simulink model "satellite"  (R2018b)
settings: Solver=VariableStepAuto  StartTime=0.0  StopTime=10.0  RelTol=1e-3
settings Model: Creator=carlos  LastModifiedBy=carlos

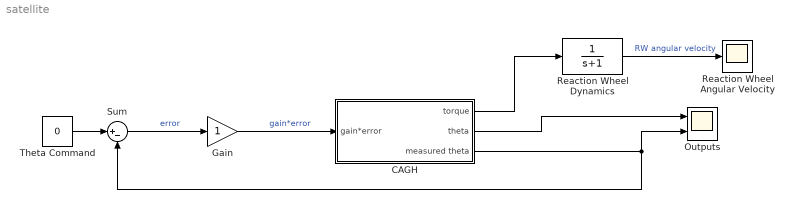
== system satellite ==
  CAGH : Subsystem
  Gain : Gain
  Outputs : Scope  NumInputPorts=2
  Reaction Wheel Angular Velocity : Scope
  Reaction Wheel Dynamics : TransferFcn  Denominator=[1 1]
  Sum : Sum  Inputs=|+-
  "Theta Command " : Constant  Value=0
  wires:
  "Theta Command "/1 -> Sum/1
  Sum/1 -> Gain/1  "error"
  Reaction Wheel Dynamics/1 -> Reaction Wheel Angular Velocity/1  "RW angular velocity"
  CAGH/3(measured theta) -> Outputs/2, Sum/2
  Gain/1 -> CAGH/1(gain*error)  "gain*error"
  CAGH/1(torque) -> Reaction Wheel Dynamics/1
  CAGH/2(theta) -> Outputs/1

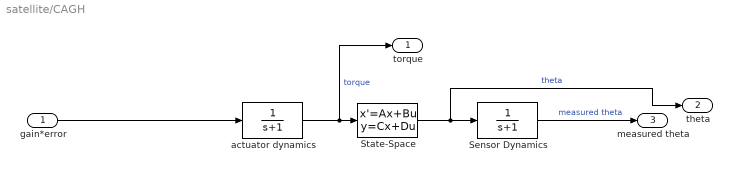
== system satellite/CAGH ==
  gain*error : Inport
  "Sensor Dynamics " : TransferFcn  Denominator=[1 1]
  State-Space : StateSpace  InitialCondition=0
  "actuator dynamics " : TransferFcn  Denominator=[1 1]
  torque : Outport
  theta : Outport  Port=2
  measured theta : Outport  Port=3
  wires:
  "Sensor Dynamics "/1 -> measured theta/1  "measured theta"
  "actuator dynamics "/1 -> torque/1, State-Space/1  "torque"
  State-Space/1 -> theta/1, "Sensor Dynamics "/1  "theta"
  gain*error/1 -> "actuator dynamics "/1
